simulink model "Actuator"  (R2023a)
settings: Solver=VariableStepAuto  StartTime=0.0  StopTime=10.0  RelTol=1e-3
undefined symbols (not defined in the file or in its folder): K, kd, ks, m, N, Td, Ti
settings Model: Creator=Sadiq Ali  LastModifiedBy=Sadiq Ali

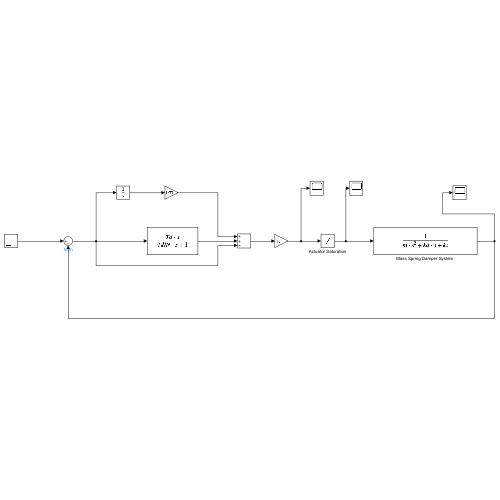
[thumbnail: Simulink's stored preview of the top-level diagram]
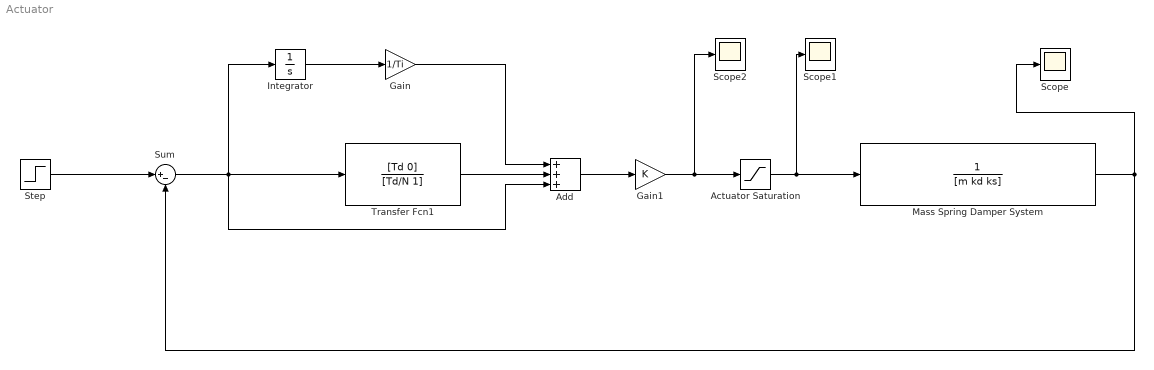
== system Actuator ==
  Actuator Saturation : Saturate  UpperLimit=50  LowerLimit=-50
  Add : Sum  Inputs=+++
  Gain : Gain  Gain=1/Ti
  Gain1 : Gain  Gain=K
  Integrator : Integrator
  "Mass Spring Damper System " : TransferFcn  Denominator=[m kd ks]
  Scope : Scope
  Scope1 : Scope
  Scope2 : Scope
  Step : Step  Time=0  SampleTime=0
  Sum : Sum  Inputs=|+-
  Transfer Fcn1 : TransferFcn  Numerator=[Td 0]  Denominator=[Td/N 1]
  wires:
  "Mass Spring Damper System "/1 -> Scope/1, Sum/2
  Step/1 -> Sum/1
  Integrator/1 -> Gain/1
  Gain/1 -> Add/1
  Transfer Fcn1/1 -> Add/2
  Sum/1 -> Add/3, Integrator/1, Transfer Fcn1/1
  Add/1 -> Gain1/1
  Gain1/1 -> Scope2/1, Actuator Saturation/1
  Actuator Saturation/1 -> Scope1/1, "Mass Spring Damper System "/1
